simulink model "hopsim2model"  (R2023b)
settings: Solver=VariableStepAuto  StartTime=0.0  StopTime=60  RelTol=1e-3
values from neighbouring files (symbols this model uses):
  G = [0 0 0     0 0 0    0 0 0    0 0 0]'    [hopsim1.m]    (also in hopsim2.m = [0 0   0 0   0 0 10    0 0 0]')
  g = 9.81    [hopsim1.m]    (also in hopsim2.m)
  K = round(K,5)    [hopsim1.m]    (also in hopsim2.m)
  l = 0.2251    [hopsim2.m]
  mass = 0.627    [hopsim1.m]    (also in hopsim2.m)
  V = 5    [hopsim1.m]    (also in hopsim2.m = 1)
libraries: shared6dof x1
settings Model: Creator=jacksonwright  LastModifiedBy=jacksonwright

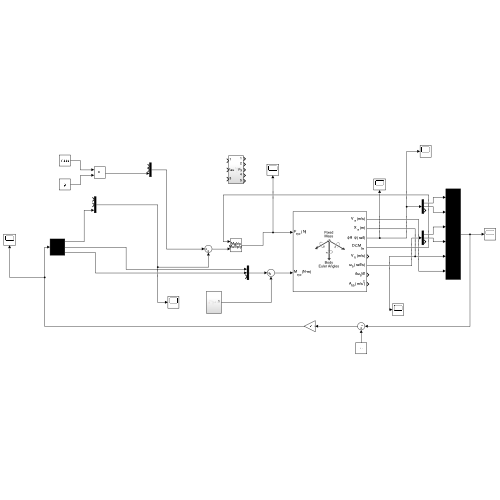
[thumbnail: Simulink's stored preview of the top-level diagram]
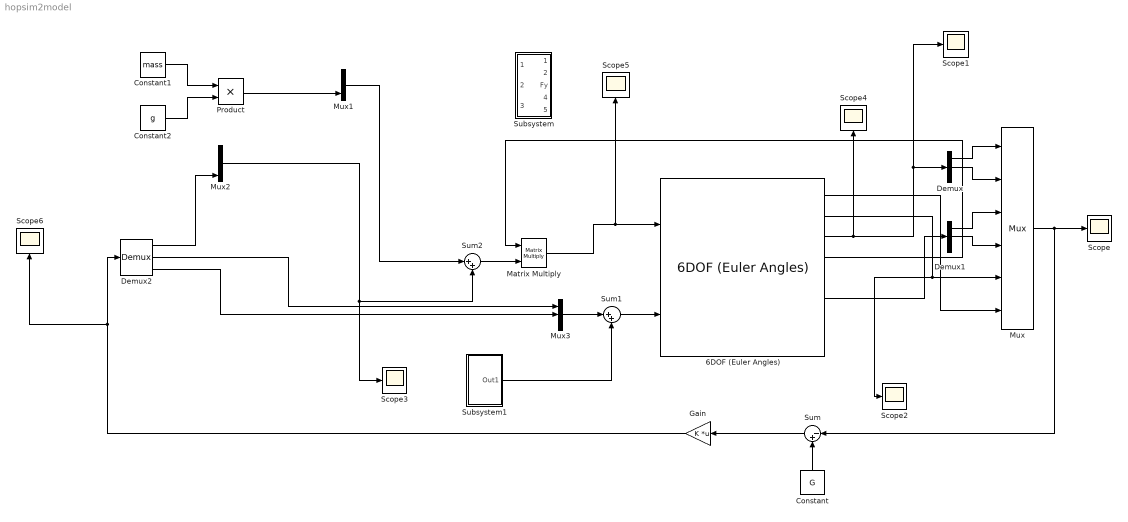
== system hopsim2model ==
  6DOF (Euler Angles) : shared6dof/6DOF (Euler Angles)  units=Metric (MKS)  mtype=Fixed  rep=Euler Angles  xme_0=[0 0 10]  Vm_0=[0 0 0]  eul_0=[0 0 0]  pm_0=[0 0 0]  mass_0=mass  mass_e=0.5  mass_f=2.0  inertia=imat  inertia_e=eye(3)  inertia_f=2*eye(3)  k_quat=1.0  vre_flag=on  abi_flag=off  aMode=0  xme_statename=''  Vm_statename=''  eul_statename=''  quat_statename=''  pm_statename=''  mass_statename=''
  Constant : Constant  Value=G
  Constant1 : Constant  Value=mass
  Constant2 : Constant  Value=g
  Demux : Demux  Outputs=3
  Demux1 : Demux  Outputs=3
  Demux2 : Demux  Outputs=3
  Gain : Gain  Gain=K  Multiplication=Matrix(K*u)
  Matrix Multiply : Product  Multiplication=Matrix(*)
  Mux : Mux  Inputs=6
  Mux1 : Mux  Inputs=3
  Mux2 : Mux  Inputs=3
  Mux3 : Mux  Inputs=3
  Product : Product
  Scope{,1..6} (7 alike) : Scope
  Subsystem : Subsystem
  Subsystem1 : Subsystem
  Sum : Sum  Inputs=|-+
  Sum1 : Sum  Inputs=|++
  Sum2 : Sum  Inputs=|++
  wires:
  6DOF (Euler Angles)/3 -> Scope4/1, Scope1/1, Demux/1
  Demux/1 -> Mux/1
  Demux/2 -> Mux/2
  6DOF (Euler Angles)/6 -> Demux1/1
  Demux1/1 -> Mux/3
  Demux1/2 -> Mux/4
  6DOF (Euler Angles)/2 -> Scope2/1, Mux/5
  6DOF (Euler Angles)/1 -> Mux/6
  Mux/1 -> Sum/1, Scope/1
  Constant/1 -> Sum/2
  Sum/1 -> Gain/1
  Gain/1 -> Scope6/1, Demux2/1
  Demux2/1 -> Mux2/3
  Mux2/1 -> Scope3/1, Sum2/2
  Subsystem1/1(Out1) -> Sum1/2
  Sum1/1 -> 6DOF (Euler Angles)/2
  6DOF (Euler Angles)/4 -> Matrix Multiply/1
  Constant1/1 -> Product/1
  Constant2/1 -> Product/2
  Mux1/1 -> Sum2/1
  Matrix Multiply/1 -> Scope5/1, 6DOF (Euler Angles)/1
  Product/1 -> Mux1/3
  Sum2/1 -> Matrix Multiply/2
  Demux2/2 -> Mux3/1
  Demux2/3 -> Mux3/2
  Mux3/1 -> Sum1/1

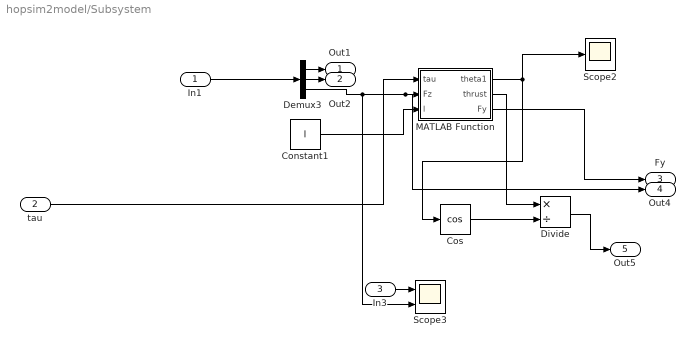
== system hopsim2model/Subsystem ==
  In1 : Inport
  tau : Inport  Port=2
  In3 : Inport  Port=3
  Constant1 : Constant  Value=l
  Cos : Trigonometry  Operator=cos
  Demux3 : Demux  Outputs=3
  Divide : Product  Inputs=*/
  MATLAB Function : MATLAB Function  TreatAsAtomicUnit=on
  Scope2 : Scope
  Scope3 : Scope  NumInputPorts=2
  Out1 : Outport
  Out2 : Outport  Port=2
  Fy : Outport  Port=3
  Out4 : Outport  Port=4
  Out5 : Outport  Port=5
  wires:
  Divide/1 -> Out5/1
  In3/1 -> Scope3/1
  MATLAB Function/3(Fy) -> Fy/1
  Demux3/1 -> Out1/1
  In1/1 -> Demux3/1
  Cos/1 -> Divide/2
  MATLAB Function/2(thrust) -> Divide/1
  Constant1/1 -> MATLAB Function/3(l)
  tau/1 -> MATLAB Function/1(tau)
  Demux3/2 -> Out2/1
  MATLAB Function/1(theta1) -> Scope2/1, Cos/1
  Demux3/3 -> Scope3/2, Out4/1, MATLAB Function/2(Fz)

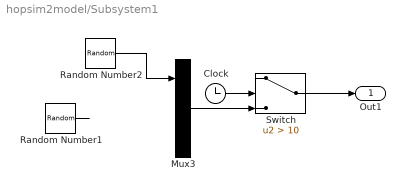
== system hopsim2model/Subsystem1 ==
  Clock : Clock
  Mux3 : Mux  Inputs=3
  Random Number1 : RandomNumber  Variance=V  SampleTime=1
  Random Number2 : RandomNumber  Variance=V  SampleTime=1
  Switch : Switch  Criteria=u2 > Threshold  Threshold=10  SaturateOnIntegerOverflow=off  InputSameDT=off
  Out1 : Outport
  wires:
  Switch/1 -> Out1/1
  Random Number2/1 -> Mux3/1
  Clock/1 -> Switch/2
  Mux3/1 -> Switch/3
  Random Number1/1 -> ?

== matlab function hopsim2model/Subsystem/MATLAB Function ==
  data: tau input; theta1 output; Fz input; l input; thrust output; Fy output
function [theta1,thrust,Fy] = fcn(tau,Fz,l)


theta1= atan(tau/(Fz*l));

thrust = Fz/cos(theta1);

Fy = thrust*sin(theta1);
